simulink model "generalized_RMLM"  (R2021b)
settings: Solver=ode23tb  StartTime=0.0  StopTime=Ts  MaxStep=1e-5  RelTol=1e-3  AbsTol=1e-3  EnableMultiTasking=on
values from neighbouring files (symbols this model uses):
  C1 = 1e-6    (= 1e-06)    [Parameter_preparation.m]    (also in TF.m)
  C2 = 180e-6    (= 0.00018)    [Parameter_preparation.m]    (also in TF.m)
  C3 = 1e-6    (= 1e-06)    [Parameter_preparation.m]    (also in TF.m)
  C4 = 100e-6    (= 0.0001)    [Parameter_preparation.m]    (also in TF.m)
  fs = 1/T/2    (= 20000)    [Parameter_preparation.m]
  L1 = 1e-6    (= 1e-06)    [Parameter_preparation.m]    (also in TF.m)
  L2 = 1e-6    (= 1e-06)    [Parameter_preparation.m]    (also in TF.m)
  Ll = 80.3e-6    (= 8.03e-05)    [TF.m]
  LM = 2600e-6    (= 0.0026)    [Parameter_preparation.m]
  n = 1/1    (= 1)    [Parameter_preparation.m]    (also in TF.m)
  R1 = 0.143    [Parameter_preparation.m]    (also in TF.m = 0.68)
  R2 = 0.094    [Parameter_preparation.m]    (also in TF.m = 0.68)
  Req = Rp + 2*Rsw + (Rs + 2*Rsw)/(n^2)    (= 0.501)    [Parameter_preparation.m]    (also in TF.m = 1.417)
  RM = 4600    [Parameter_preparation.m]    (also in TF.m = 2000)
  Ro = 20    [Parameter_preparation.m]    (also in TF.m = 0.5)
  Ts = 0.7    [Parameter_preparation.m]
  Vin = 100    [Parameter_preparation.m]    (also in TF.m)
  Vo = 0    [Parameter_preparation.m]    (also in TF.m)
undefined symbols (not defined in the file or in its folder): plecs
libraries: slpidlib x1
settings Model: Creator=Kai  LastModifiedBy=Administrator
settings SolverCC: AutoScaleAbsTol=off  AlgebraicLoopSolver=TrustRegion
settings DataIOCC: FinalStateName=xFinal_avg  InitialState=xFinal_avg  SaveFormat=Array  SignalLoggingSaveFormat=ModelDataLogs  ReturnWorkspaceOutputs=off  TimeSaveName=tout_avg  OutputSaveName=yout_avg
settings OptimizationCC: ExpressionDepthLimit=2147483647  LifeSpan=inf
settings DebuggingCC: UnderspecifiedInitializationDetection=Classic  MergeDetectMultiDrivingBlocksExec=none  SolverPrmCheckMsg=warning  MultiTaskDSMMsg=warning  MultiTaskCondExecSysMsg=none  StateNameClashWarn=warning  SFUnexpectedBacktrackingDiag=warning  SFNoUnconditionalDefaultTransitionDiag=warning  SFExecutionAtInitializationDiag=none  SFMachineParentedDataDiag=warning  ArithmeticOperatorsInVariantConditions=warning
settings HardwareCC: ProdBitPerPointer=32  ProdBitPerSizeT=32  ProdBitPerPtrDiffT=32  ProdLargestAtomicFloat=None  ProdIntDivRoundTo=Undefined  ProdEndianess=Unspecified  ProdWordSize=32  ProdHWDeviceType=32-bit Generic
settings ModelReferenceCC: PropagateSignalLabelsOutOfModel=off
settings SFSimCC: SimUseLocalCustomCode=off  CustomCodeUndefinedFunction=UseInterfaceOnly
settings RTWCC: RTWUseLocalCustomCode=off
settings CodeAppCC: StateflowObjectComments=on
settings GRTTargetCC: TargetLangStandard=C89/C90 (ANSI)
settings ConfigComp: CovMetricSettings=dw  CovSaveCumulativeToWorkspaceVar=on  CovSaveSingleToWorkspaceVar=on  CovExternalEMLEnable=off

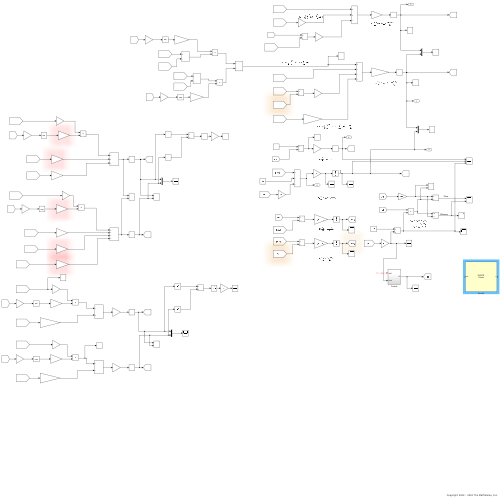
[thumbnail: Simulink's stored preview of the top-level diagram]
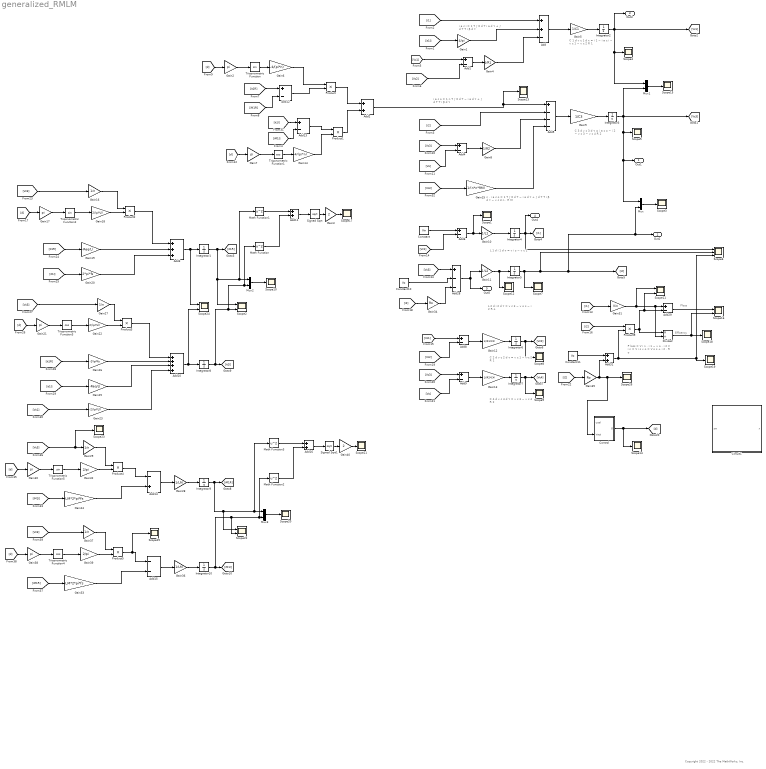
== system generalized_RMLM ==
  note: i a c o = 1 n T ∫ 0 d T − i α d τ + ∫ d T T i β d τ
  note: i a c i = 1 T ∫ 0 d T i α d τ + ∫ d T T i β d τ
  note: P loss = V i n ⋅ i 1 − v o ⋅ i 2 V i n = V i s v o = V o s + i 2 ⋅ R o
  note: C 3 d v c 3 d τ = i a c o − i 2 − v c 3 − v c 4 R 2
  note: n ⋅ i a c o = 1 T ∫ 0 d T − i α d τ + ∫ d T T i β d τ − v c 3 n ⋅ R M
  note: C 1 d v c 1 d τ = i 1 − i a c i − v c 1 − v c 2 R 1
  note: L 1 d i 1 d τ = v i s − v c 1
  note: L 2 d i 2 d τ = v c 3 − v o s − i 2 R o
  note: C 2 d v c 2 d τ = v c 1 − v c 2 R 1
  note: C 4 d v c 4 d τ = v c 3 − v c 4 R 2
  note: Efficency
  note: Ploss
  note: Copyright 2022 - 2022 The MathWorks, Inc.
  Add : Sum  Inputs=++-
  Add{1,4,6,8..9,12..13,29} (8 alike) : Sum  Inputs=+-
  Add10 : Sum  Inputs=++++
  Add{2,11,16,31} (4 alike) : Sum
  Add14 : Sum  Inputs=-+
  Add15 : Sum  Inputs=--
  Add28 : Sum  Inputs=+--
  Add3 : Sum  Inputs=+++
  Add5 : Sum  Inputs=+---
  Circuit1 : Subsystem  LoadFcn=plecs('sl', 200);  InitFcn=plecs('sl', 214);  StartFcn=plecs('sl', 208);  StopFcn=plecs('sl', 209);  mask(PlecsCircuit){REPLACE_WITH_PLECS_VAR=REPLACE_WITH_PLECSCIRCUIT_CODE, PLECSData=<binary blob, 3212 chars, not shown>}
      mask prompts: REPLACE_WITH_PLECS_VAR "PLECS Data (Do not delete or modify!)"; PLECSData "PLECS Data (Do not delete or modify!)"
      mask init:
      | % PLACE CUSTOM INITIALIZATIONS ABOVE
      | % DO NOT REMOVE
      | plecs('sl', 215);
      | % DO NOT REMOVE
      settings: CopyFcn=plecs('sl', 203);  DeleteFcn=plecs('sl', 205);  UndoDeleteFcn=plecs('sl', 206);  PreSaveFcn=plecs('sl', 211);  PostSaveFcn=plecs('sl', 201);  NameChangeFcn=plecs('sl', 210);  DestroyFcn=plecs('sl', 207);  PreCopyFcn=plecs('sl', 216);  OpenFcn=plecs('sl', 202);  ErrorFcn=plerrorfcn
      mask Help: web(['file:///' fullfile(plecsdoc, 'creatingacircuit.html')])
      mask Display: disp('PLECS\nCircuit')
  Constant : Constant  Value=Vin
  Constant10 : Constant  Value=Vo
  Constant11 : Constant  Value=Vo
  Control : Subsystem
  Divide2 : Product  Inputs=*/
  Gain1 : Gain  Gain=4/pi
  Gain10 : Gain  Gain=1/L1
  Gain11 : Gain  Gain=1/L2
  Gain12 : Gain  Gain=1/(R1*C2)
  Gain13 : Gain  Gain=1/(R2*C4)
  Gain14 : Gain  Gain=-4/(pi*n)
  Gain15 : Gain  Gain=1/(n*n*RM)
  Gain{16,27,29,37} (4 alike) : Gain  Gain=1/n
  Gain{2,7,17,21,30,38} (6 alike) : Gain  Gain=pi
  Gain18 : Gain  Gain=2/(pi*Ll)
  Gain19 : Gain  Gain=-Req/Ll
  Gain20 : Gain  Gain=2*pi*fs
  Gain22 : Gain  Gain=2/(pi*Ll)
  Gain23 : Gain  Gain=-2/(pi*Ll)
  Gain24 : Gain  Gain=LM*2*pi*fs
  Gain25 : Gain  Gain=-Req/Ll
  Gain26 : Gain  Gain=-2*pi*fs
  Gain28 : Gain  Gain=1/LM
  Gain3 : Gain  Gain=2
  Gain31 : Gain  Gain=Vin
  Gain32 : Gain  Gain=2/pi
  Gain33 : Gain  Gain=LM*2*pi*fs
  Gain34 : Gain  Gain=Ro
  Gain35 : Gain  Gain=Ro
  Gain36 : Gain  Gain=1/LM
  Gain39 : Gain  Gain=2/pi
  Gain4 : Gain  Gain=1/R1
  Gain40 : Gain  Gain=2
  Gain5 : Gain  Gain=1/C1
  Gain6 : Gain  Gain=-4/(pi*n)
  Gain8 : Gain  Gain=1/R2
  Gain9 : Gain  Gain=1/C3
  Integrator{1,4..5,8..10} (6 alike) : Integrator
  Integrator2 : Integrator  InitialCondition=Vin
  Integrator3 : Integrator  InitialCondition=Vo
  Integrator6 : Integrator  InitialCondition=Vin
  Integrator7 : Integrator  InitialCondition=Vo
  Math Function{,1..3} (4 alike) : Math  Operator=square  SignedPower=on  SaturateOnIntegerOverflow=on
  Mux{,1..3} (4 alike) : Mux  Inputs=2
  Product{,1..5,9} (7 alike) : Product  RndMeth=Zero
  Scope{1,3..5,7..10,12..15,17..21,23,25..26} (20 alike) : Scope
  Scope{2,11,16,22,24} (5 alike) : Scope  NumInputPorts=2
  Scope6 : Scope  NumInputPorts=3
  Signed Sqrt : Sqrt  SaturateOnIntegerOverflow=on
  Signed Sqrt1 : Sqrt  SaturateOnIntegerOverflow=on
  Trigonometric Function : Trigonometry
  Trigonometric Function1 : Trigonometry  Operator=cos
  Trigonometric Function2 : Trigonometry
  Trigonometric Function3 : Trigonometry  Operator=cos
  Trigonometric Function4 : Trigonometry  Operator=cos
  Trigonometric Function5 : Trigonometry
  Out1 : Outport
  Out2 : Outport  Port=2
  Out3 : Outport  Port=3
  Out4 : Outport  Port=4
  Out5 : Outport  Port=5
  wires:
  Constant/1 -> Add6/1
  Add6/1 -> Scope1/1, Gain10/1
  Gain10/1 -> Integrator4/1
  Integrator4/1 -> Out4/1, Scope6/1, [i1]
  Add28/1 -> Gain11/1, Out5/1
  Gain11/1 -> Scope12/1, Integrator5/1
  Integrator5/1 -> Scope6/2, Out2/1, Mux/2, [i2], Scope7/1
  [Vc2] -> Add8/2
  Add8/1 -> Gain12/1
  Gain12/1 -> Integrator6/1
  Integrator6/1 -> Scope8/1, [Vc2]
  [Vc3] -> Add9/1
  [Vo] -> Add9/2
  Add9/1 -> Gain13/1
  Gain13/1 -> Integrator7/1
  Integrator7/1 -> Scope9/1, [Vc4]
  [Vc2] -> Add1/2
  Add1/1 -> Gain4/1
  Add/1 -> Gain5/1
  [Vc3] -> Add4/1
  [Vo] -> Add4/2
  Add4/1 -> Gain8/1
  Add5/1 -> Gain9/1
  Gain9/1 -> Integrator3/1
  [it1I] -> Gain1/1
  Gain8/1 -> Add5/3
  [i2] -> Add5/2
  Mux/1 -> Scope3/1
  Mux1/1 -> Scope15/1
  Integrator2/1 -> [Vc1], Out3/1, Mux1/1, Scope4/1
  Integrator3/1 -> [Vc3], Mux1/2, Scope5/1, Out1/1, Mux/1
  [Vc3] -> Add28/1
  Constant10/1 -> Add28/2
  [Vc1] -> Add1/1
  [Vc1] -> Add6/2
  [Vc1] -> Add8/1
  [i1] -> Gain31/1
  [i2] -> Product9/1
  Gain31/1 -> Scope11/1, Divide2/2, Add29/1
  Product9/1 -> Scope11/2, Add29/2, Divide2/1
  Add29/1 -> Scope16/1
  Divide2/1 -> Scope16/2, Scope18/1
  [i2] -> Gain34/1
  Gain34/1 -> Add28/3
  Constant11/1 -> Add31/1
  Add31/1 -> Product9/2, Scope19/1, Scope6/3
  [d] -> Gain2/1
  Gain2/1 -> Trigonometric Function/1
  Trigonometric Function/1 -> Gain6/1
  [d] -> Gain7/1
  Gain7/1 -> Trigonometric Function1/1
  Trigonometric Function1/1 -> Gain14/1
  Product/1 -> Add2/1
  Product1/1 -> Add2/2
  Add2/1 -> Scope13/1, Add5/1
  Gain6/1 -> Product/1
  Gain14/1 -> Product1/2
  [d] -> Gain17/1
  Gain17/1 -> Trigonometric Function2/1
  Trigonometric Function2/1 -> Gain18/1
  Gain18/1 -> Product2/2
  [it1R] -> Gain19/1
  [it1I] -> Gain20/1
  Gain19/1 -> Add3/2
  Gain20/1 -> Add3/3
  Product2/1 -> Add3/1
  Add3/1 -> Scope24/1, Integrator1/1
  Integrator1/1 -> Math Function1/1, Mux2/1, Scope2/1, [it1R]
  [d] -> Gain21/1
  Gain21/1 -> Trigonometric Function3/1
  Trigonometric Function3/1 -> Gain22/1
  Gain22/1 -> Product3/2
  [it1R] -> Gain26/1
  [it1I] -> Gain25/1
  Product3/1 -> Add10/1
  Gain25/1 -> Add10/3
  Gain26/1 -> Add10/2
  Gain23/1 -> Add10/4
  [Vc1] -> Gain23/1
  Mux2/1 -> Scope10/1
  Integrator8/1 -> Math Function/1, Mux2/2, Scope2/2, [it1I]
  Add11/1 -> Signed Sqrt/1
  Signed Sqrt/1 -> Gain3/1
  Gain3/1 -> Scope17/1
  Math Function1/1 -> Add11/1
  Math Function/1 -> Add11/2
  [i1] -> Add/1
  Gain4/1 -> Add/3
  Gain5/1 -> Integrator2/1
  Gain1/1 -> Add/2
  [it1R] -> Add12/1
  Add12/1 -> Product/2
  [it1I] -> Add13/1
  Add13/1 -> Product1/1
  [Vc3] -> Gain15/1
  Gain15/1 -> Add5/4
  Gain16/1 -> Product2/1
  Gain27/1 -> Product3/1
  [d] -> Gain30/1
  Gain30/1 -> Trigonometric Function5/1
  Trigonometric Function5/1 -> Gain32/1
  Gain32/1 -> Product4/2
  Gain29/1 -> Product4/1
  [iM1I] -> Gain24/1
  Product4/1 -> Add14/1
  Gain24/1 -> Add14/2
  Add14/1 -> Gain28/1
  Gain28/1 -> Integrator9/1
  [d] -> Gain38/1
  Gain38/1 -> Trigonometric Function4/1
  Trigonometric Function4/1 -> Gain39/1
  Gain39/1 -> Product5/2
  Gain37/1 -> Product5/1
  [iM1R] -> Gain33/1
  Product5/1 -> Scope25/1, Add15/1
  Gain33/1 -> Add15/2
  Add15/1 -> Gain36/1
  Gain36/1 -> Integrator10/1
  Integrator9/1 -> Scope22/1, Mux3/1, Math Function3/1, [iM1R]
  Mux3/1 -> Scope20/1
  Integrator10/1 -> Scope22/2, Mux3/2, Math Function2/1, [iM1I]
  Add16/1 -> Signed Sqrt1/1
  Signed Sqrt1/1 -> Gain40/1
  Gain40/1 -> Scope21/1
  Math Function3/1 -> Add16/1
  Math Function2/1 -> Add16/2
  [Vc3] -> Scope23/1, Gain29/1
  [Vc3] -> Gain37/1
  [Vc3] -> Gain27/1
  [Vc3] -> Gain16/1
  Add10/1 -> Scope24/2, Integrator8/1
  [iM1R] -> Add12/2
  [iM1I] -> Add13/2
  [i2] -> Gain35/1
  ? -> Control/1(Vref)
  Control/1(G) -> Scope14/1, [d]
  Gain35/1 -> Control/2(Vout), Scope26/1, Add31/2

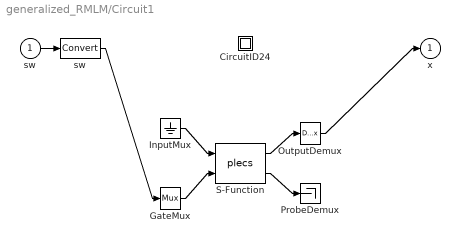
== system generalized_RMLM/Circuit1 ==
  sw : Inport  PortDimensions=8
  " CircuitID24 " : Subsystem
  " GateMux " : Mux  Inputs=[ 8 ]
  " InputMux " : Ground
  " OutputDemux " : Demux  Outputs=[ 1 ]
  " ProbeDemux " : Terminator
  " S-Function " : S-Function  FunctionName=plecs  SFunctionDeploymentMode=off  EnableBusSupport=off
  " sw " : DataTypeConversion  SaturateOnIntegerOverflow=on  RndMeth=Zero
  x : Outport  PortDimensions=1
  wires:
  " InputMux "/1 -> " S-Function "/1
  " GateMux "/1 -> " S-Function "/2
  " S-Function "/1 -> " OutputDemux "/1
  " S-Function "/2 -> " ProbeDemux "/1
  sw/1 -> " sw "/1
  " sw "/1 -> " GateMux "/1
  " OutputDemux "/1 -> x/1

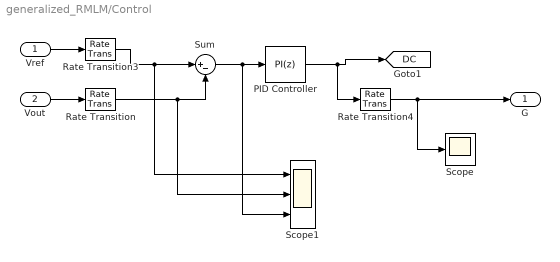
== system generalized_RMLM/Control ==
  Vref : Inport
  Vout : Inport  Port=2
  PID Controller : slpidlib/PID Controller  Controller=PI  Form=Parallel  TimeDomain=Discrete-time  UseExternalTs=off  SampleTime=Ts  IntegratorMethod=Forward Euler  FilterMethod=Forward Euler  ControllerParametersSource=internal  P=0.018311  I=312.0658  D=0  UseFilter=on  N=106819.177082171  TunerSelectOption=Transfer Function Based (PID Tuner App)  InitialConditionSource=internal  InitialConditionForIntegrator=0  InitialConditionForFilter=0  DifferentiatorICPrevScaledInput=0  ExternalReset=none  TrackingMode=off  Kt=1  LimitOutput=off  SatLimitsSource=internal  UpperSaturationLimit=inf  LowerSaturationLimit=-inf  LinearizeAsGain=on  AntiWindupMode=none  Kb=1  POutMin=[]  POutMax=[]  IOutMin=[]  IOutMax=[]  DOutMin=[]  DOutMax=[]  NOutMin=[]  NOutMax=[]  SumOutMin=[]  SumOutMax=[]  SaturationOutMin=[]  SaturationOutMax=[]  PParamMin=[]  PParamMax=[]  IParamMin=[]  IParamMax=[]  DParamMin=[]  DParamMax=[]  NParamMin=[]  NParamMax=[]  KbParamMin=[]  KbParamMax=[]  KtParamMin=[]  KtParamMax=[]  KbOutMin=[]  KbOutMax=[]  KtOutMin=[]  KtOutMax=[]  IntegratorOutMin=[]  IntegratorOutMax=[]  FilterOutMin=[]  FilterOutMax=[]  SumI1OutMin=[]  SumI1OutMax=[]  SumI2OutMin=[]  SumI2OutMax=[]  SumI3OutMin=[]  SumI3OutMax=[]  SumI4OutMin=[]  SumI4OutMax=[]  SumDOutMin=[]  SumDOutMax=[]  DifferentiatorOutMin=[]  DifferentiatorOutMax=[]  FilterDiffOutCoefMin=[]  FilterDiffOutCoefMax=[]  ReciprocalOutMin=[]  ReciprocalOutMax=[]  SumDenOutMin=[]  SumDenOutMax=[]  SumNumOutMin=[]  SumNumOutMax=[]  DivideOutMin=[]  DivideOutMax=[]  UdiffTsProdOutMin=[]  UdiffTsProdOutMax=[]  NTsProdOutMin=[]  NTsProdOutMax=[]  UintegralTsProdOutMin=[]  UintegralTsProdOutMax=[]  UngainTsProdOutMin=[]  UngainTsProdOutMax=[]  IntegratorContinuousStateAttributes=''  IntegratorStateMustResolveToSignalObject=off  IntegratorRTWStateStorageClass=Auto  FilterContinuousStateAttributes=''  FilterStateMustResolveToSignalObject=off  FilterRTWStateStorageClass=Auto  ParallelPVariant=InternalParameters  IdealPVariant=Disabled  IVariant=InternalParameters  DVariant=Disabled  IntegratorVariant=Discrete  SatVariant=Disabled  AWVariant=Passthrough  PCopyVariant=Disabled  TRVariant=Disabled  FdbkBlocksVariant=Forward  IdealPFdbkVariant=Disabled  SatFdbkVariant=Disabled  DerivativeFilterVariant=Disabled  NVariant=Disabled  NCopyVariant=Disabled_SignalSpec  FilterICVariant=Disabled  IntegratorICVariant=InternalICs  ExternalResetVariant=Disabled  TRSumVariant=Passthrough  SumFdbkVariant=Disabled  SumVariant=Sum_PI  TsampFilterVariant=InternalTs  TsampNgainVariant=Passthrough  TsampIntegralVariant=Passthrough  ExternalSaturationOutDataTypeStr=Inherit: Same as second input
  Rate Transition : RateTransition  OutPortSampleTime=5e-8
  Rate Transition3 : RateTransition  OutPortSampleTime=5e-8
  Rate Transition4 : RateTransition
  Scope : Scope
  Scope1 : Scope  NumInputPorts=3
  Sum : Sum  Inputs=|+-
  G : Outport  VectorParamsAs1DForOutWhenUnconnected=off
  tag scope: DC=global
  wires:
  Vref/1 -> Rate Transition3/1
  Rate Transition3/1 -> Scope1/1, Sum/1
  Vout/1 -> Rate Transition/1
  Rate Transition4/1 -> Scope/1, G/1
  Sum/1 -> Scope1/3, PID Controller/1
  PID Controller/1 -> Rate Transition4/1, [DC]
  Rate Transition/1 -> Scope1/2, Sum/2

== system generalized_RMLM/Circuit1/ CircuitID24  ==
